simulink model "Exercise_2_2_1_Nonlinear_Quaternions_new"  (R2021a)
settings: Solver=VariableStepAuto  StartTime=0.0  StopTime=simTime  RelTol=1e-3
values from neighbouring files (symbols this model uses):
  b = 0.001    [Exercise_2_Workspace.mat]
  D = [0.01  0  0; 0  0.01  0; 0  0  0.01]    [Exercise_2_Workspace.mat]
  g = [0 0 -9.81]    [Exercise_2_Workspace.mat]
  k = 0.01    [Exercise_2_Workspace.mat]
  L = 0.225    [Exercise_2_Workspace.mat]
  m = 0.5    [Exercise_2_Workspace.mat]
  MoI = [3e-06  0  0; 0  3e-06  0; 0  0  1e-05]    [Exercise_2_Workspace.mat]
  omega = [0 0 0]    [Exercise_2_Workspace.mat]
  p = [0 0 0]    [Exercise_2_Workspace.mat]
  p_dot = [0 0 0]    [Exercise_2_Workspace.mat]
  quaternion = [1 0 0 0]    [Exercise_2_Workspace.mat]
  RPM = [0 1000 0 1000]    [Exercise_2_Workspace.mat]
  TakeStep = 1    [Exercise_2_Workspace.mat]
undefined symbols (not defined in the file or in its folder): Newton, Raphson
settings Model: Creator=Wojciech  LastModifiedBy=Wojciech

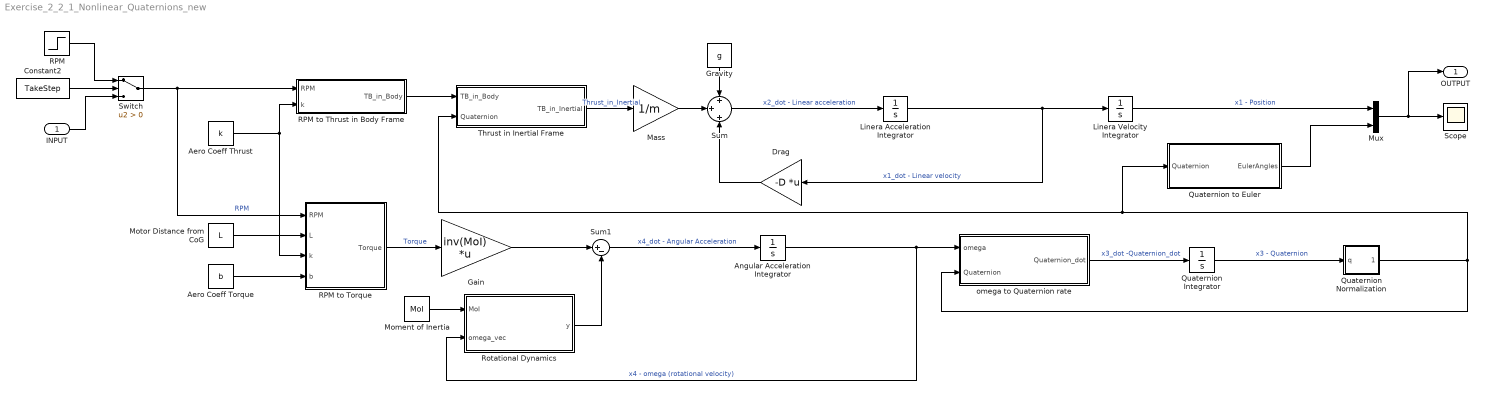
== system Exercise_2_2_1_Nonlinear_Quaternions_new ==
  INPUT : Inport  PortDimensions=4
  Aero Coeff Thrust : Constant  Value=k
  Aero Coeff Torque : Constant  Value=b
  Angular Acceleration Integrator : Integrator  Priority=4  InitialCondition=omega
  Constant2 : Constant  Value=TakeStep
  Drag : Gain  Gain=-D  Multiplication=Matrix(K*u)
  Gain : Gain  Gain=inv(MoI)  Multiplication=Matrix(K*u)
  Gravity : Constant  Value=g  VectorParams1D=off
  Linera Acceleration Integrator : Integrator  Priority=2  InitialCondition=p_dot
  Linera Velocity Integrator : Integrator  Priority=1  InitialCondition=p
  Mass : Gain  Gain=1/m
  Moment of Inertia : Constant  Value=MoI  VectorParams1D=off
  Motor Distance from CoG : Constant  Value=L
  Mux : Mux  Inputs=2
  Quaternion Normalization : Subsystem
  Quaternion Integrator : Integrator  Priority=3  InitialCondition=quaternion
  Quaternion to Euler : MATLAB Function  TreatAsAtomicUnit=on
  RPM : Step  Time=0  After=RPM  SampleTime=0
  RPM to Thrust in Body Frame : MATLAB Function  TreatAsAtomicUnit=on
  RPM to Torque : MATLAB Function  TreatAsAtomicUnit=on
  Rotational Dynamics : MATLAB Function  TreatAsAtomicUnit=on
  Scope : Scope
  Sum : Sum  Inputs=+|+|+
  Sum1 : Sum  Inputs=|+-
  Switch : Switch  Criteria=u2 > Threshold
  Thrust in Inertial Frame : MATLAB Function  TreatAsAtomicUnit=on
  omega to Quaternion rate : MATLAB Function  TreatAsAtomicUnit=on
  OUTPUT : Outport
  wires:
  Linera Velocity Integrator/1 -> Mux/1  "x1 - Position"
  Linera Acceleration Integrator/1 -> Drag/1, Linera Velocity Integrator/1  "x1_dot - Linear velocity"
  Sum/1 -> Linera Acceleration Integrator/1  "x2_dot - Linear acceleration"
  Gravity/1 -> Sum/1
  RPM to Thrust in Body Frame/1(TB_in_Body) -> Thrust in Inertial Frame/1(TB_in_Body)
  Aero Coeff Thrust/1 -> RPM to Thrust in Body Frame/2(k), RPM to Torque/3(k)
  Thrust in Inertial Frame/1(TB_in_Inertial) -> Mass/1  "Thrust_in_Inertial"
  Mass/1 -> Sum/2
  Drag/1 -> Sum/3
  Motor Distance from CoG/1 -> RPM to Torque/2(L)
  Aero Coeff Torque/1 -> RPM to Torque/4(b)
  RPM to Torque/1(Torque) -> Gain/1  "Torque"
  Gain/1 -> Sum1/1
  Rotational Dynamics/1(y) -> Sum1/2
  Moment of Inertia/1 -> Rotational Dynamics/1(MoI)
  Sum1/1 -> Angular Acceleration Integrator/1  "x4_dot - Angular Acceleration"
  Angular Acceleration Integrator/1 -> omega to Quaternion rate/1(omega), Rotational Dynamics/2(omega_vec)  "x4 - omega (rotational velocity)"
  omega to Quaternion rate/1(Quaternion_dot) -> Quaternion Integrator/1  "x3_dot -Quaternion_dot"
  Quaternion Integrator/1 -> Quaternion Normalization/1(q)  "x3 - Quaternion"
  Mux/1 -> OUTPUT/1, Scope/1
  Constant2/1 -> Switch/2
  INPUT/1 -> Switch/3
  RPM/1 -> Switch/1
  Switch/1 -> RPM to Thrust in Body Frame/1(RPM), RPM to Torque/1(RPM)  "RPM"
  Quaternion to Euler/1(EulerAngles) -> Mux/2
  Quaternion Normalization/1(qnorm) -> Quaternion to Euler/1(Quaternion), Thrust in Inertial Frame/2(Quaternion), omega to Quaternion rate/2(Quaternion)

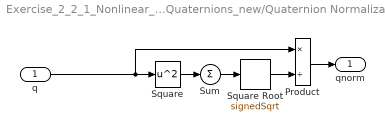
== system Exercise_2_2_1_Nonlinear_Quaternions_new/Quaternion Normalization ==
  q : Inport  PortDimensions=4
  Product : Product  Inputs=*/  InputSameDT=on  RndMeth=Zero  SaturateOnIntegerOverflow=on  OutDataTypeStr=Inherit: Same as first input
  Square : Math  Operator=square  SignedPower=on  SaturateOnIntegerOverflow=on
  Square Root : Sqrt  Operator=signedSqrt  AlgorithmType=Newton-Raphson  SaturateOnIntegerOverflow=on
  Sum : Sum  Inputs=1  InputSameDT=on  SaturateOnIntegerOverflow=on  OutDataTypeStr=Inherit: Same as first input
  qnorm : Outport  PortDimensions=4
  wires:
  Product/1 -> qnorm/1
  Square Root/1 -> Product/2
  Square/1 -> Sum/1
  Sum/1 -> Square Root/1
  q/1 -> Product/1, Square/1

== matlab function Exercise_2_2_1_Nonlinear_Quaternions_new/RPM to Thrust in Body Frame ==
  data: RPM input; TB_in_Body output; k input
function TB_in_Body = fcn(RPM, k)
TB_in_Body = k * [0; 0; RPM'*RPM];

== matlab function Exercise_2_2_1_Nonlinear_Quaternions_new/Thrust in Inertial Frame ==
  data: TB_in_Body input; Quaternion input; TB_in_Inertial output
function TB_in_Inertial = fcn(TB_in_Body, Quaternion)

q0 = Quaternion(1);
q1 = Quaternion(2);
q2 = Quaternion(3);
q3 = Quaternion(4);

%transforming a quaternion into a direction cosine matrix [DCM] R
R = [   q0^2 + q1^2 - q2^2 - q3^2, 2*(q1*q2 + q3*q0), 2*(q1*q3 - q2*q0);
        2*(q1*q2 - q3*q0), q0^2 - q1^2 + q2^2 - q3^2, 2*(q2*q3 + q1*q0);
        2*(q1*q3 + q2*q0), 2*(q2*q3 - q1*q0), q0^2 - q1^2 - q2^2 + q3^2];

TB_in_Inertial = R * TB_in_Body;

== matlab function Exercise_2_2_1_Nonlinear_Quaternions_new/RPM to Torque ==
  data: RPM input; Torque output; L input; k input; b input
function Torque = fcn(RPM, L, k, b)

Torque = [  L*k*(RPM(1)^2 - RPM(3)^2); ...
            L*k*(RPM(2)^2 - RPM(4)^2); ...
            b * (RPM(1)^2 - RPM(2)^2 + RPM(3)^2 - RPM(4)^2)];

== matlab function Exercise_2_2_1_Nonlinear_Quaternions_new/Rotational Dynamics ==
  data: MoI input; omega_vec input; y output
function y = fcn(MoI, omega_vec)
Ixx = MoI(1,1);
Iyy = MoI(2,2);
Izz = MoI(3,3);

omega_x = omega_vec(1);
omega_y = omega_vec(2);
omega_z = omega_vec(3);

y = [ (Iyy-Izz)/Ixx*omega_y*omega_z; ...
      (Izz-Ixx)/Iyy*omega_x*omega_z; ...
      (Ixx-Iyy)/Izz*omega_x*omega_y];

== matlab function Exercise_2_2_1_Nonlinear_Quaternions_new/omega to Quaternion rate ==
  data: omega input; Quaternion_dot output; Quaternion input
function Quaternion_dot = fcn(omega, Quaternion)

omega_quat = [0; omega];

q0 = Quaternion(1);
q1 = Quaternion(2);
q2 = Quaternion(3);
q3 = Quaternion(4);

B = [   q0, -q1, -q2, -q3;
        q1, q0, -q3, q2;
        q2, q3, q0, -q1;
        q3, -q2, q1, q0];
  
Quaternion_dot = 0.5 * B * omega_quat;

== matlab function Exercise_2_2_1_Nonlinear_Quaternions_new/Quaternion to Euler ==
  data: Quaternion input; EulerAngles output
function EulerAngles = fcn(Quaternion)

q0 = Quaternion(1);
q1 = Quaternion(2);
q2 = Quaternion(3);
q3 = Quaternion(4);

% two step procedure
% firstly converting quaternion into direction cosine matrix [DCM] R

R = [   q0^2 + q1^2 - q2^2 - q3^2, 2*(q1*q2 + q3*q0), 2*(q1*q3 - q2*q0);
        2*(q1*q2 - q3*q0), q0^2 - q1^2 + q2^2 - q3^2, 2*(q2*q3 + q1*q0);
        2*(q1*q3 + q2*q0), 2*(q2*q3 - q1*q0), q0^2 - q1^2 - q2^2 + q3^2];
    
% secondly converting R to Euler angles

phi     = atan(R(3,2) / R(3,3));
theta   = -asin(R(3,1));
psi     = atan(R(2,1) / R(1,1));

EulerAngles = [phi, theta, psi]';
